simulink model "heater"  (R2025b)
settings: Solver=VariableStepAuto  StartTime=0.0  StopTime=10.0  RelTol=1e-3
settings Model: Creator=hahnc  LastModifiedBy=hahnc

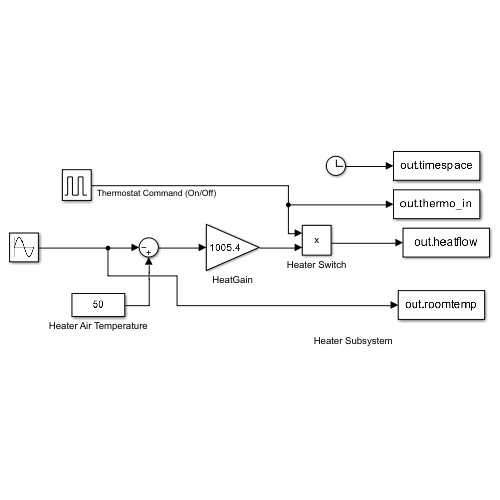
[thumbnail: Simulink's stored preview of the top-level diagram]
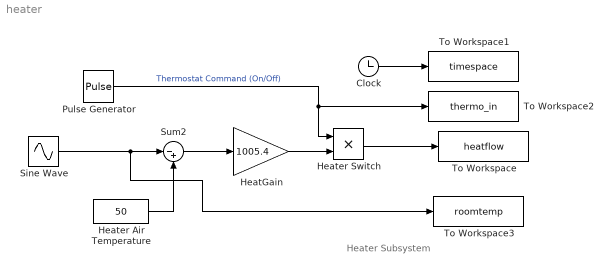
== system heater ==
  note: Heater Subsystem
  Clock : Clock
  HeatGain : Gain  Gain=1005.4
  Heater Air Temperature : Constant  Value=50
  Heater Switch : Product  RndMeth=Zero
  Pulse Generator : DiscretePulseGenerator  PulseType=Time based  Period=5  PulseWidth=50
  Sine Wave : Sin  Amplitude=15  Bias=50  SampleTime=0
  Sum2 : Sum  Inputs=|-+
  To Workspace : ToWorkspace  VariableName=heatflow  SampleTime=-1
  To Workspace1 : ToWorkspace  VariableName=timespace  SampleTime=-1
  To Workspace2 : ToWorkspace  VariableName=thermo_in  SampleTime=-1
  To Workspace3 : ToWorkspace  VariableName=roomtemp  SampleTime=-1
  wires:
  Sum2/1 -> HeatGain/1
  Pulse Generator/1 -> To Workspace2/1, Heater Switch/1  "Thermostat Command (On/Off)"
  HeatGain/1 -> Heater Switch/2
  Heater Air Temperature/1 -> Sum2/2
  Clock/1 -> To Workspace1/1
  Sine Wave/1 -> To Workspace3/1, Sum2/1
  Heater Switch/1 -> To Workspace/1
